simulink model "Fig328"  (R2014b)
settings: Solver=ode3  StartTime=0.0  StopTime=3  FixedStep=2e-6  RelTol=1e-5
libraries: commfilt2 x2, commutil2 x1, commchan3 x1, commanapbnd3 x1, commrandsrc2 x1
settings Model: Creator=Dennis Silage  LastModifiedBy=Silage
settings DataIOCC: SignalLoggingSaveFormat=ModelDataLogs
settings OptimizationCC: ExpressionDepthLimit=2147483647  InitFltsAndDblsToZero=on
settings DebuggingCC: UnderspecifiedInitializationDetection=Classic  MergeDetectMultiDrivingBlocksExec=none  SolverPrmCheckMsg=none  FcnCallInpInsideContextMsg=UseLocalSettings  StateNameClashWarn=warning
settings GRTTargetCC: CombineOutputUpdateFcns=off  GRTInterface=on

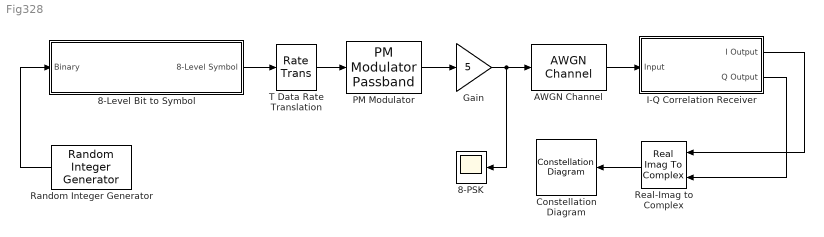
== system Fig328 ==
  "8-Level Bit to Symbol " : Subsystem
  8-PSK : Scope
      settings: TimeRange=0.005  YMin=-6  YMax=6
  AWGN Channel : commchan3/AWGN Channel  InputProcessing=Inherited (this choice will be removed - see release notes)  seed=randseed  noiseMode="Signal to noise ratio  (Eb/No)"  EbNodB=15  EsNodB=20  SNRdB=10  bitsPerSym=3  Ps=12.5  Tsym=3e-3  variance=0
  Constellation Diagram : ConstellationDiagram
  Gain : Gain  Gain=5
  I-Q Correlation Receiver : Subsystem
  PM Modulator : commanapbnd3/PM Modulator Passband  Fc=20000  Ph=0  Kc=pi/4
  Random Integer Generator : commrandsrc2/Random Integer Generator  mul=2  seed=randseed  Ts=1e-3  frameBased=off  sampPerFrame=1  orient=off  outDataType=double
  Real-Imag to Complex : RealImagToComplex
  T Data Rate Translation : RateTransition  OutPortSampleTime=2e-6
  wires:
  AWGN Channel/1 -> I-Q Correlation Receiver/1(Input)
  Gain/1 -> AWGN Channel/1, 8-PSK/1
  T Data Rate Translation/1 -> PM Modulator/1
  PM Modulator/1 -> Gain/1
  Random Integer Generator/1 -> "8-Level Bit to Symbol "/1(Binary)
  "8-Level Bit to Symbol "/1(8-Level Symbol) -> T Data Rate Translation/1
  Real-Imag to Complex/1 -> Constellation Diagram/1
  I-Q Correlation Receiver/1(I Output) -> Real-Imag to Complex/1
  I-Q Correlation Receiver/2(Q Output) -> Real-Imag to Complex/2

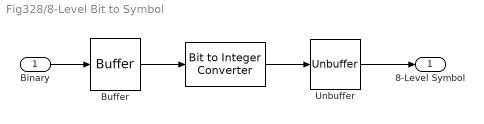
== system Fig328/8-Level Bit to Symbol  ==
  Binary : Inport
  " " : commutil2/Bit to Integer Converter  nbits=3  bitOrder=MSB first  signedOutputValues=Unsigned  outDtype=Inherit via internal rule  outDtypeSigned=Inherit via internal rule
  Buffer : Buffer  N=3  TreatMby1Signals=One channel
  Unbuffer : Unbuffer  ic=3  SampleBasedProcessing=Same as frame based
  8-Level Symbol : Outport
  wires:
  Binary/1 -> Buffer/1
  Buffer/1 -> " "/1
  " "/1 -> Unbuffer/1
  Unbuffer/1 -> 8-Level Symbol/1

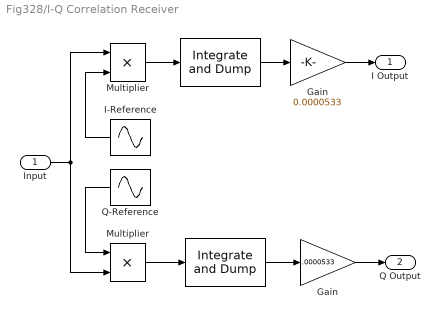
== system Fig328/I-Q Correlation Receiver ==
  Input : Inport
  " " : commfilt2/Integrate and Dump  obssamples=1500  offsetsamples=0  nodump=off  roundingMode=Floor  overflowMode=off
  "  " : commfilt2/Integrate and Dump  obssamples=1500  offsetsamples=0  nodump=off  roundingMode=Floor  overflowMode=off
  Gain : Gain  Gain=0.0000533
  "Gain " : Gain  Gain=.0000533
  I-Reference : Sin  Amplitude=5  Frequency=40000*pi  Phase=pi/2  SampleTime=2e-6
  Multiplier : Product  RndMeth=Zero
  "Multiplier " : Product  RndMeth=Zero
  Q-Reference : Sin  Amplitude=5  Frequency=40000*pi  SampleTime=2e-6
  I Output : Outport
  Q Output : Outport  Port=2
  wires:
  "Multiplier "/1 -> " "/1
  Multiplier/1 -> "  "/1
  I-Reference/1 -> "Multiplier "/2
  Q-Reference/1 -> Multiplier/1
  Input/1 -> "Multiplier "/1, Multiplier/2
  " "/1 -> Gain/1
  "  "/1 -> "Gain "/1
  Gain/1 -> I Output/1
  "Gain "/1 -> Q Output/1
